simulink model "LowPass"  (R2022a)
settings: Solver=VariableStepAuto  StartTime=0.0  StopTime=inf  RelTol=1e-3
InitFcn:
  | Ts=0.001;
  | L_G=1;
  | 
  | n = 200; % Number of nodes (original 100)
  | k = 10;   % Degree of each node (each node connects to 6 others)
  | 
  | % Initialize the adjacency matrix with zeros
  | A = zeros(n);
  | 
  | % Fill the adjacency matrix (ring lattice structure)
  | for i = 1:n
  |     for j = 1:k/2
  |         A(i, mod(i+j-1, n) + 1) = 1;
  |         A(i, mod(i-j-1, n) + 1) = 1;
  |     end
  | end
  | 
  | % Since the graph is undirected, A is symmetric
  | A = (A + A') > 0;
  | A =double(A); % Convert logical to double
  | % Create the degree matrix
  | D = k * eye(n);
  | % Compute the Laplacian matrix
  | L = L_G*(D - A);
settings Model: Creator=syedabuz  LastModifiedBy=Lirui
settings ModelReferenceCC: EnableRefExpFcnMdlSchedulingChecks=off
settings RTWCC: Description=Generic Real-Time Target

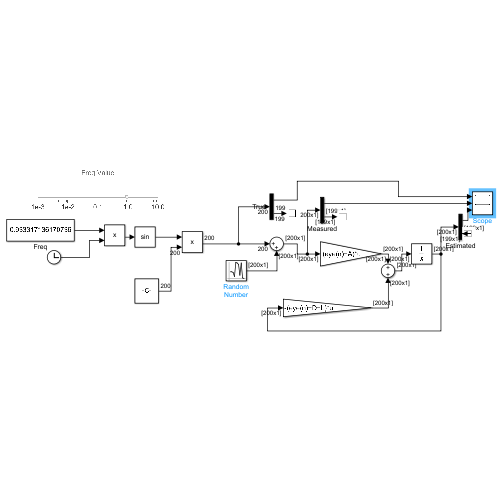
[thumbnail: Simulink's stored preview of the top-level diagram]
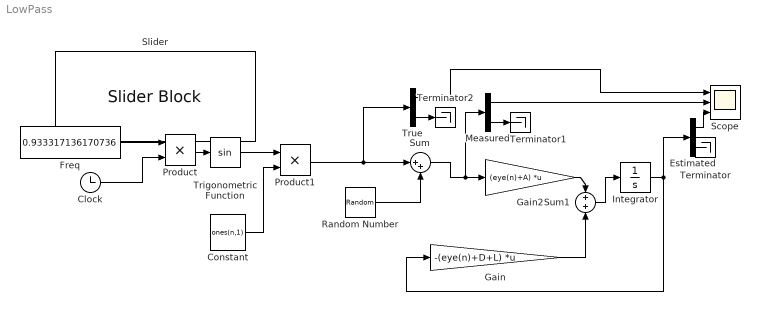
== system LowPass ==
  Clock : Clock
  Constant : Constant  Value=ones(n,1)
  Estimated : Demux  Outputs=[1 n-1]
  Freq : Constant  Value=0.933317136170736
  Gain : Gain  Gain=-(eye(n)+D+L)  Multiplication=Matrix(K*u)
  Gain2 : Gain  Gain=(eye(n)+A)  Multiplication=Matrix(K*u)
  Integrator : Integrator
  Measured : Demux  Outputs=[1 n-1]
  Product : Product
  Product1 : Product
  Random Number : RandomNumber  Mean=0.0*ones(n,1)  Variance=0.3*ones(n,1)  Seed=[1:n]'-50  SampleTime=Ts  VectorParams1D=off
  Scope : Scope  NumInputPorts=3
  Slider : SliderBlock  ScaleMin=0.001  ScaleMax=10  ScaleType=Log
  Sum : Sum  Inputs=|++
  Sum1 : Sum
  Terminator : Terminator
  Terminator1 : Terminator
  Terminator2 : Terminator
  Trigonometric Function : Trigonometry
  True : Demux  Outputs=[1 n-1]
  wires:
  Product1/1 -> Sum/1, True/1
  Random Number/1 -> Sum/2
  Gain2/1 -> Sum1/1
  Gain/1 -> Sum1/2
  Sum1/1 -> Integrator/1
  Integrator/1 -> Estimated/1, Gain/1
  Sum/1 -> Measured/1, Gain2/1
  Estimated/2 -> Terminator/1
  Estimated/1 -> Scope/3
  Measured/2 -> Terminator1/1
  Measured/1 -> Scope/2
  True/2 -> Terminator2/1
  True/1 -> Scope/1
  Product/1 -> Trigonometric Function/1
  Clock/1 -> Product/2
  Freq/1 -> Product/1
  Constant/1 -> Product1/2
  Trigonometric Function/1 -> Product1/1
